simulink model "simulation_sm_WP1"  (R2023a)
settings: Solver=VariableStepAuto  StartTime=0.0  StopTime=20  RelTol=1e-3
values from neighbouring files (symbols this model uses):
  K = [18235, 53.9]    [u_definition_WP1.m]
  kr = 18235    [u_definition_WP1.m]
settings Model: Creator=miche  LastModifiedBy=miche

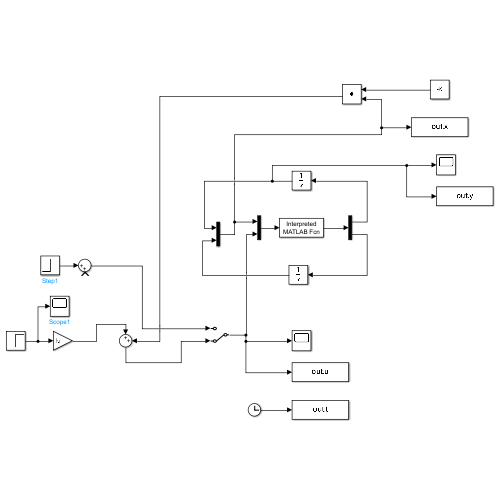
[thumbnail: Simulink's stored preview of the top-level diagram]
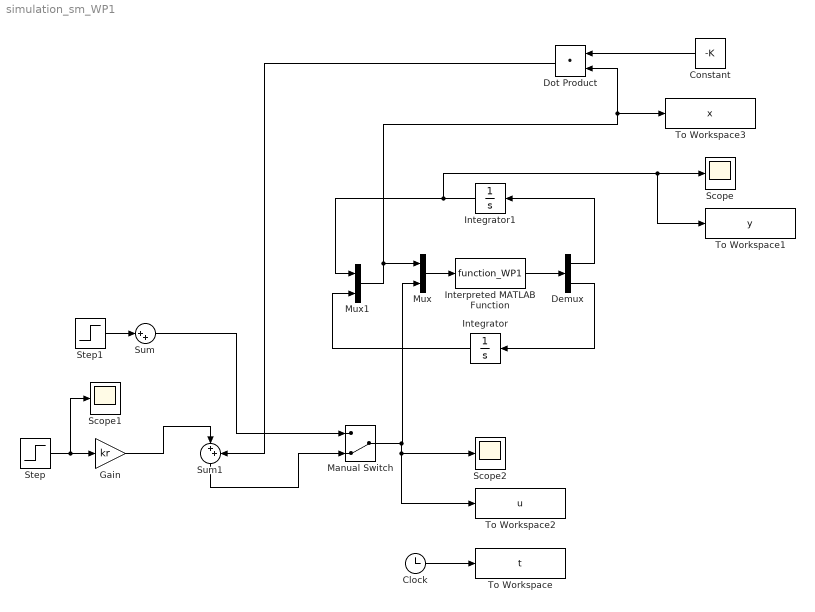
== system simulation_sm_WP1 ==
  Clock : Clock
  Constant : Constant  Value=-K
  Demux : Demux  Outputs=2
  Dot Product : DotProduct  OutDataTypeStr=Inherit: Inherit via internal rule
  Gain : Gain  Gain=kr
  Integrator : Integrator
  Integrator1 : Integrator
  Interpreted MATLAB Function : MATLABFcn  MATLABFcn=function_WP1  OutputDimensions=2
  Manual Switch : ManualSwitch  CurrentSetting=0
  Mux : Mux  Inputs=2
  Mux1 : Mux  Inputs=2
  Scope : Scope
  Scope1 : Scope
  Scope2 : Scope
  Step : Step  After=pi  SampleTime=0
  Step1 : Step  Time=10  SampleTime=0
  Sum : Sum  Inputs=|++
  Sum1 : Sum  Inputs=|++
  To Workspace : ToWorkspace  VariableName=t  SampleTime=-1
  To Workspace1 : ToWorkspace  VariableName=y  SampleTime=-1
  To Workspace2 : ToWorkspace  VariableName=u  SampleTime=-1
  To Workspace3 : ToWorkspace  VariableName=x  SampleTime=-1
  wires:
  Clock/1 -> To Workspace/1
  Step/1 -> Scope1/1, Gain/1
  Constant/1 -> Dot Product/1
  Mux/1 -> Interpreted MATLAB Function/1
  Interpreted MATLAB Function/1 -> Demux/1
  Demux/2 -> Integrator/1
  Integrator1/1 -> To Workspace1/1, Scope/1, Mux1/1
  Integrator/1 -> Mux1/2
  Demux/1 -> Integrator1/1
  Mux1/1 -> Dot Product/2, To Workspace3/1, Mux/1
  Gain/1 -> Sum1/1
  Dot Product/1 -> Sum1/2
  Step1/1 -> Sum/1
  Manual Switch/1 -> Mux/2, To Workspace2/1, Scope2/1
  Sum1/1 -> Manual Switch/2
  Sum/1 -> Manual Switch/1
